simulink model "Practica1_DoblePSim"  (R2022b)
settings: Solver=ode45  StartTime=0.0  StopTime=10.0  FixedStep=0.00001  MaxStep=0.00001  RelTol=1e-3
values from neighbouring files (symbols this model uses):
  g = 9.81    [Practica1_DobleP.m]
  l1 = 0.3    [Practica1_DobleP.m]
  l2 = 0.25    [Practica1_DobleP.m]
  m1 = 0.2    [Practica1_DobleP.m]
  m2 = 0.1    [Practica1_DobleP.m]
settings Model: Creator=mluser  LastModifiedBy=Alan

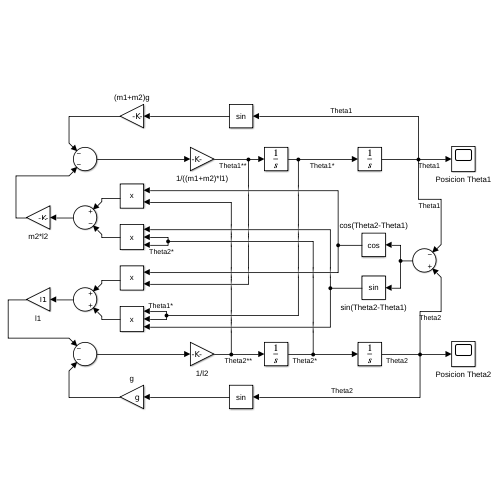
[thumbnail: Simulink's stored preview of the top-level diagram]
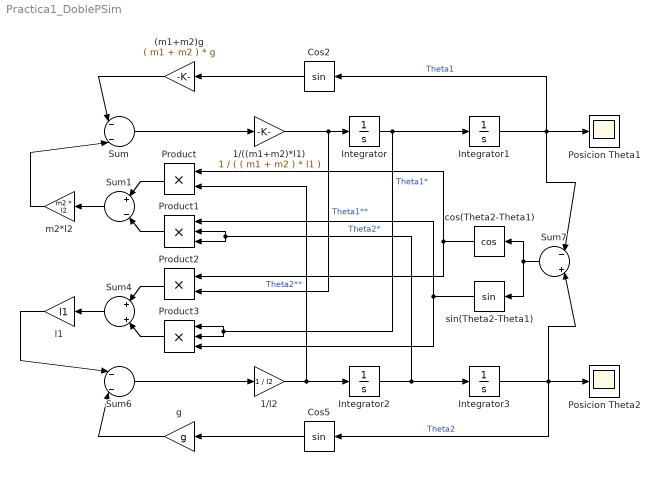
== system Practica1_DoblePSim ==
  (m1+m2)g : Gain  Gain=( m1 + m2 ) * g
  1/((m1+m2)*l1) : Gain  Gain=1 / ( ( m1 + m2 ) * l1 )
  1/l2 : Gain  Gain=1 / l2
  Cos2 : Trigonometry
  Cos5 : Trigonometry
  Integrator : Integrator
  Integrator1 : Integrator
  Integrator2 : Integrator
  Integrator3 : Integrator  InitialCondition=(35 * pi) / 180
  Posicion Theta1 : Scope
  Posicion Theta2 : Scope
  Product : Product
  Product1 : Product  Inputs=3
  Product2 : Product
  Product3 : Product  Inputs=3
  Sum : Sum  Inputs=|-|-|
  Sum1 : Sum  Inputs=|+|-|
  Sum4 : Sum  Inputs=|+|+|
  Sum6 : Sum  Inputs=|-|-|
  Sum7 : Sum  Inputs=|-|+|
  cos(Theta2-Theta1) : Trigonometry  Operator=cos
  g : Gain  Gain=g
  l1 : Gain  Gain=l1
  m2*l2 : Gain  Gain=m2 * l2
  sin(Theta2-Theta1) : Trigonometry
  wires:
  1/((m1+m2)*l1)/1 -> Product2/2, Integrator/1  "Theta1**"
  Sum/1 -> 1/((m1+m2)*l1)/1
  Integrator/1 -> Integrator1/1, Product3/1, Product3/2  "Theta1*"
  Integrator1/1 -> Cos2/1, Sum7/1, Posicion Theta1/1  "Theta1"
  m2*l2/1 -> Sum/2
  Product/1 -> Sum1/1
  Sum1/1 -> m2*l2/1
  1/l2/1 -> Integrator2/1, Product/2  "Theta2**"
  Integrator2/1 -> Integrator3/1, Product1/2, Product1/3  "Theta2*"
  Cos2/1 -> (m1+m2)g/1
  (m1+m2)g/1 -> Sum/1
  Sum4/1 -> l1/1
  cos(Theta2-Theta1)/1 -> Product2/1, Product/1
  Product2/1 -> Sum4/1
  sin(Theta2-Theta1)/1 -> Product1/1, Product3/3
  Product3/1 -> Sum4/2
  Sum6/1 -> 1/l2/1
  Cos5/1 -> g/1
  Sum7/1 -> sin(Theta2-Theta1)/1, cos(Theta2-Theta1)/1
  Integrator3/1 -> Cos5/1, Posicion Theta2/1, Sum7/2  "Theta2"
  Product1/1 -> Sum1/2
  l1/1 -> Sum6/1
  g/1 -> Sum6/2
